simulink model "Modelo_da_Planta_Linear"  (R2018b)
settings: Solver=ode4  StartTime=0.0  StopTime=100  FixedStep=0.002  RelTol=1e-3
libraries: simulink x1
settings Model: Creator=pedro  LastModifiedBy=pedro
settings SFSimCC: SimUseLocalCustomCode=off
settings RTWCC: RTWUseLocalCustomCode=off
settings CodeAppCC: StateflowObjectComments=on

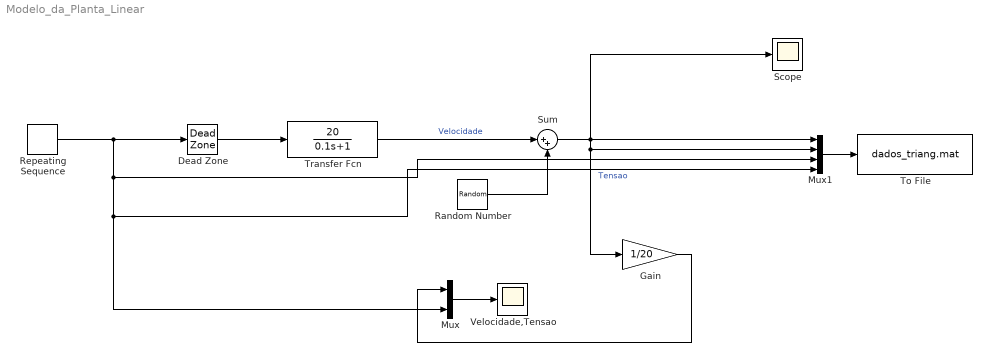
== system Modelo_da_Planta_Linear ==
  Dead Zone : DeadZone  LowerValue=-1.2  SaturateOnIntegerOverflow=on
  Gain : Gain  Gain=1/20
  Mux : Mux  Inputs=2
  Mux1 : Mux
  Random Number : RandomNumber  SampleTime=0.1
  Repeating Sequence : simulink/Sources/Repeating Sequence  rep_seq_t=[0 1 2 3 4]  rep_seq_y=[0 5 0 -5 0]
  Scope : Scope
  Sum : Sum  Inputs=|++
  To File : ToFile  Filename=dados_triang.mat  MatrixName=dados
  Transfer Fcn : TransferFcn  Numerator=[20]  Denominator=[0.1 1]
  Velocidade,Tensao : Scope
  wires:
  Repeating Sequence/1 -> Dead Zone/1, Mux1/3, Mux1/4, Mux/2  "Tensao"
  Dead Zone/1 -> Transfer Fcn/1
  Transfer Fcn/1 -> Sum/1  "Velocidade"
  Mux/1 -> Velocidade,Tensao/1
  Sum/1 -> Mux1/1, Mux1/2, Gain/1, Scope/1
  Random Number/1 -> Sum/2
  Gain/1 -> Mux/1
  Mux1/1 -> To File/1
